simulink model "Hardware_Code"  (R2025b)
settings: Solver=FixedStepAuto  StartTime=0.0  StopTime=30  RelTol=1e-3  EnableMultiTasking=on
InitFcn:
  | battery_init;
  | Full_Charge_Volt=4.2; % unit volts
  | Cutoff_Volt=3; % unit volts
  | Delta=.02;
  | ContactorTime=20;
  | ContactorTimeOut=100;
  | High_TempLim=333;
  | Low_TempLim=253;
  | Sensor_Fault_Treshold=.02;
  | CurrentTimeout=1;
  | Allowed_Delta=.04;
  | Bal_On_Time=30;
  | Bal_Off_Time=5;
  | BalNotAct_Time=10;
values from neighbouring files (symbols this model uses):
  Charge_Rate = 1    [battery_init.m]
  Discharge_Rate = -1    [battery_init.m]
  Fly_Cycle_Current = [ ... (first row only)    [battery_init.m]
undefined symbols (not defined in the file or in its folder): batt, From_Plant_MATLABStruct, SRE
libraries: fl_lib x69, nesl_utility x54, ee_lib x12, batteryecm_lib x12, simulink x6, BatteryCurrentManagement x1
(part 1 of 2)
settings Model: DataDictionary=Needed_Buses.sldd  Creator=Odonata-KJ  LastModifiedBy=Odonata-KJ
settings OptimizationCC: DefaultParameterBehavior=Inlined  EnhancedBackFolding=on  PassReuseOutputArgsAs=Individual arguments  ZeroExternalMemoryAtStartup=off  ZeroInternalMemoryAtStartup=off  MaxStackSize=64  OptimizeBlockOrder=speed  DifferentSizesBufferReuse=on  OptimizationCustomize=off  EfficientTunableParamExpr=on
settings DebuggingCC: ParameterPrecisionLossMsg=none  ParameterTunabilityLossMsg=error  BusObjectLabelMismatch=none
settings HardwareCC: ProdBitPerPointer=32.0  ProdBitPerSizeT=32.0  ProdBitPerPtrDiffT=32.0  ProdLargestAtomicInteger=Long  ProdLargestAtomicFloat=Double  ProdWordSize=32.0  ProdLongLongMode=on  ProdHWDeviceType=ARM Compatible->ARM Cortex-M
settings SFSimCC: MATLABDynamicMemAlloc=off
settings RTWCC: SystemTargetFile=ert.tlc  HardwareBoard=STM32F4xx Based  TemplateMakefile=ert_default_tmf  Toolchain=GNU Tools for ARM Embedded Processors  Description=Embedded Coder
settings CodeAppCC: ForceParamTrailComments=on  IgnoreCustomStorageClasses=off  OperatorAnnotations=on  SimulinkDataObjDesc=on  SFDataObjDesc=on  InsertBlockDesc=on
settings ERTTargetCC: ExtModeTransport=3.0  ExtModeStaticAlloc=on  ExtModeStaticAllocSize=2048.0  ExtModeMexFile=ext_xcp  ExtModeIntrfLevel=Level2 - Open  TargetLangStandard=C99 (ISO)  CodeReplacementLibrary=ARM Cortex-M

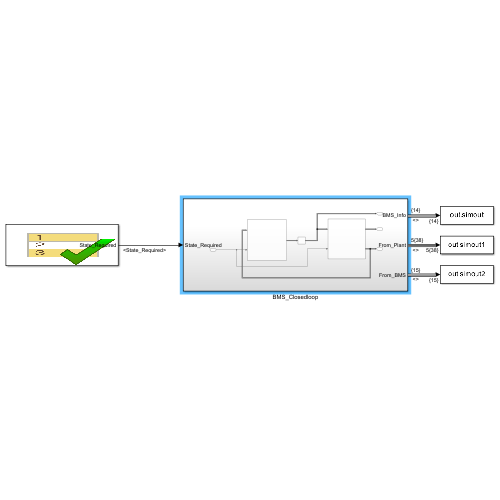
[thumbnail: Simulink's stored preview of the top-level diagram]
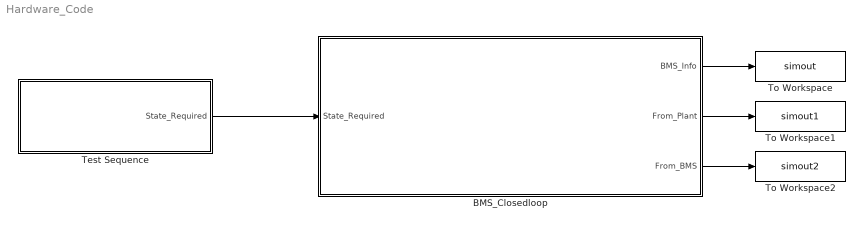
== system Hardware_Code ==
  BMS_Closedloop : Subsystem
  Test Sequence : Test Sequence  TreatAsAtomicUnit=on
  To Workspace : ToWorkspace  VariableName=simout  SaveFormat=Timeseries  SampleTime=-1
  To Workspace1 : ToWorkspace  VariableName=simout1  SaveFormat=Timeseries  SampleTime=-1
  To Workspace2 : ToWorkspace  VariableName=simout2  SaveFormat=Timeseries  SampleTime=-1
  wires:
  Test Sequence/1(State_Required) -> BMS_Closedloop/1(State_Required)
  BMS_Closedloop/1(BMS_Info) -> To Workspace/1
  BMS_Closedloop/2(From_Plant) -> To Workspace1/1
  BMS_Closedloop/3(From_BMS) -> To Workspace2/1

== system Hardware_Code/BMS_Closedloop ==
  State_Required : Inport
  BMS_Control : Subsystem
  Plant : Subsystem
  Unit Delay1 : UnitDelay  InitialCondition=From_Plant_MATLABStruct  SampleTime=-1  HasFrameUpgradeWarning=on
  BMS_Info : Outport
  From_Plant : Outport  Port=2
  From_BMS : Outport  Port=3
  wires:
  BMS_Control/1(BMS_Info) -> BMS_Info/1
  State_Required/1 -> BMS_Control/2(State_Required), Plant/2(State_Required)
  Plant/1(From_Plant) -> Unit Delay1/1
  BMS_Control/2(From_BMS) -> Plant/1(From_BMS), From_BMS/1
  Unit Delay1/1 -> From_Plant/1, BMS_Control/1(From_Plant)

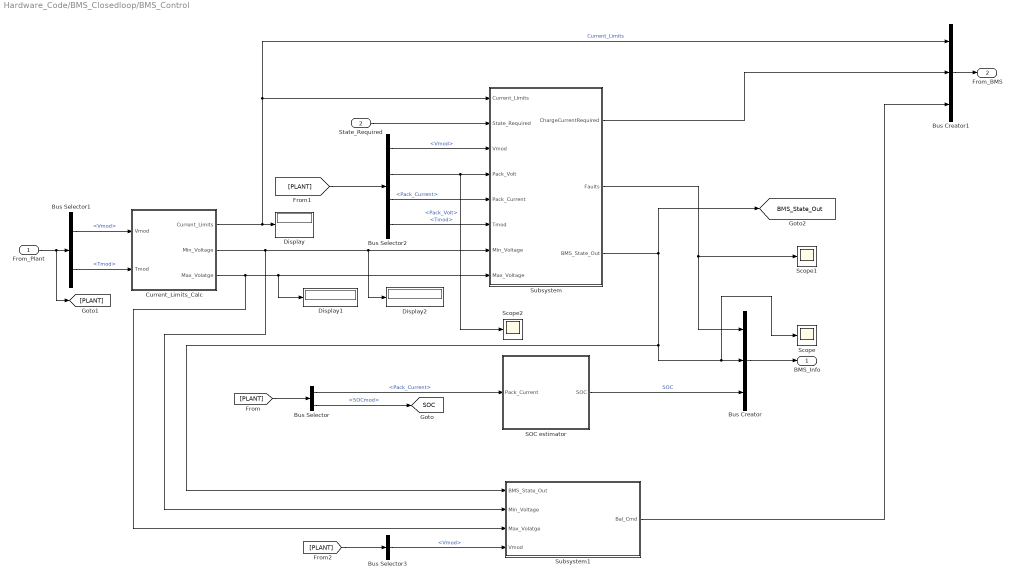
== system Hardware_Code/BMS_Closedloop/BMS_Control ==
  From_Plant : Inport
  State_Required : Inport  Port=2
  Bus Creator : BusCreator  Inputs=3
  Bus Creator1 : BusCreator  Inputs=3
  Bus Selector : BusSelector  OutputSignals=Pack_Current,SOCmod
  Bus Selector1 : BusSelector  OutputSignals=Vmod,Tmod
  Bus Selector2 : BusSelector  OutputSignals=Vmod,Pack_Volt,Pack_Current,Tmod
  Bus Selector3 : BusSelector  OutputSignals=Vmod
  Current_Limits_Calc : Subsystem
  Display : Display
  Display1 : Display
  Display2 : Display
  SOC estimator : Subsystem
  Scope : Scope
      settings: ActiveDisplayYMinimum=-0.83098117909981006  ActiveDisplayYMaximum=3.72716725840019  DataLoggingVariableName=ScopeData6
  Scope1 : Scope
      settings: ActiveDisplayYMinimum=-2.061290929652265  ActiveDisplayYMaximum=1.5304217223919956  DataLoggingVariableName=ScopeData7
  Scope2 : Scope
      settings: ActiveDisplayYMinimum=-21.052574610728009  ActiveDisplayYMaximum=61.397323890688391  DataLoggingVariableName=ScopeData8
  Subsystem : Subsystem
  Subsystem1 : Subsystem
  BMS_Info : Outport
  From_BMS : Outport  Port=2
  tag scope: BMS_State_Out=global, SOC=global
  wires:
  From_Plant/1 -> [PLANT], Bus Selector1/1
  [PLANT] -> Bus Selector/1
  Bus Selector1/1 -> Current_Limits_Calc/1(Vmod)  "<Vmod>"
  Current_Limits_Calc/2(Min_Voltage) -> Display2/1, Subsystem/7(Min_Voltage), Subsystem1/2(Min_Voltage)
  Current_Limits_Calc/3(Max_Volatge) -> Subsystem/8(Max_Voltage), Display1/1, Subsystem1/3(Max_Volatge)
  Current_Limits_Calc/1(Current_Limits) -> Subsystem/1(Current_Limits), Bus Creator1/1, Display/1  "Current_Limits"
  State_Required/1 -> Subsystem/2(State_Required)
  SOC estimator/1(SOC) -> Bus Creator/3  "SOC"
  Bus Creator/1 -> BMS_Info/1
  [PLANT] -> Bus Selector2/1
  Bus Creator1/1 -> From_BMS/1
  Subsystem/1(ChargeCurrentRequired) -> Bus Creator1/2
  Subsystem/2(Faults) -> Scope1/1, Bus Creator/1
  Subsystem/3(BMS_State_Out) -> [BMS_State_Out], Subsystem1/1(BMS_State_Out), Scope/1, Bus Creator/2
  [PLANT] -> Bus Selector3/1
  Bus Selector3/1 -> Subsystem1/4(Vmod)  "<Vmod>"
  Subsystem1/1(Bal_Cmd) -> Bus Creator1/3
  Bus Selector/1 -> SOC estimator/1(Pack_Current)  "<Pack_Current>"
  Bus Selector/2 -> [SOC]  "<SOCmod>"
  Bus Selector2/1 -> Subsystem/3(Vmod)  "<Vmod>"
  Bus Selector2/4 -> Subsystem/6(Tmod)  "<Tmod>"
  Bus Selector2/2 -> Scope2/1, Subsystem/4(Pack_Volt)  "<Pack_Volt>"
  Bus Selector2/3 -> Subsystem/5(Pack_Current)  "<Pack_Current>"
  Bus Selector1/2 -> Current_Limits_Calc/2(Tmod)  "<Tmod>"

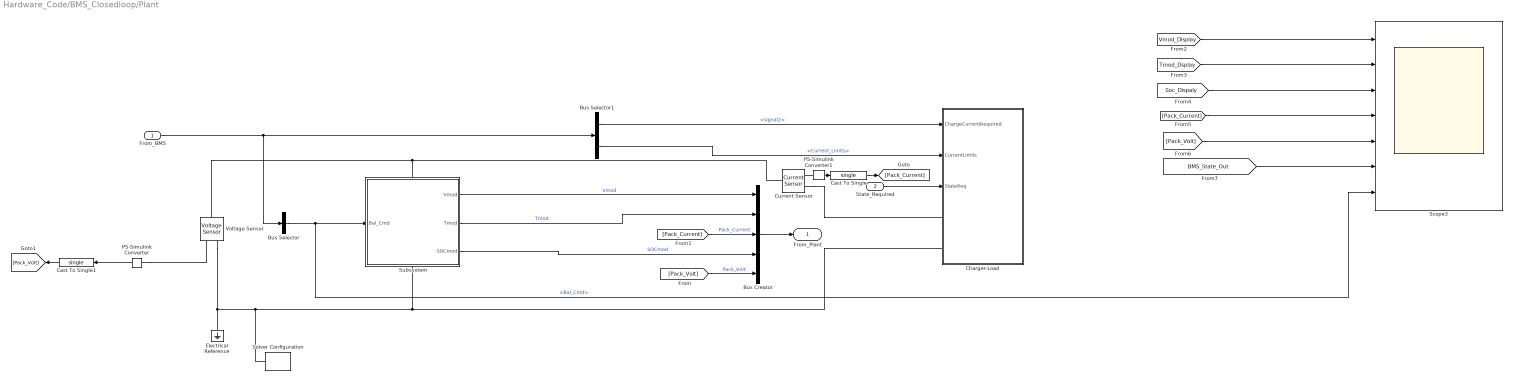
== system Hardware_Code/BMS_Closedloop/Plant ==
  From_BMS : Inport
  State_Required : Inport  Port=2
  Bus Creator : BusCreator  Inputs=5
  Bus Selector : BusSelector  OutputSignals=Bal_Cmd
  Bus Selector1 : BusSelector  OutputSignals=signal2,Current_Limits
  Cast To Single : DataTypeConversion  OutDataTypeStr=single  SaturateOnIntegerOverflow=off  RndMeth=Floor
  Cast To Single1 : DataTypeConversion  OutDataTypeStr=single  SaturateOnIntegerOverflow=off  RndMeth=Floor
  Charger-Load : Subsystem
  Current Sensor : fl_lib/Electrical/Electrical Sensors/Current Sensor
  Electrical Reference : fl_lib/Electrical/Electrical Elements/Electrical Reference
  PS-Simulink Converter : nesl_utility/PS-Simulink Converter  PhysicalDomain=network_engine_domain  SubClassName=ps_output  LeftPortType=input  RightPortType=output  PseudoPeriodic=off  Frequencies=[]  VectorFormat=inherit  Unit=inherit  AffineConversion=off
  PS-Simulink Converter1 : nesl_utility/PS-Simulink Converter  PhysicalDomain=network_engine_domain  SubClassName=ps_output  LeftPortType=input  RightPortType=output  PseudoPeriodic=off  Frequencies=[]  VectorFormat=inherit  Unit=inherit  AffineConversion=off
  Scope3 : Scope  NumInputPorts=7
      settings: ActiveDisplayString=5  ActiveDisplayYMinimum=32.848355293273926  ActiveDisplayYMaximum=53.971850395202637  YLabel=Pack Volt  DataLoggingVariableName=ScopeData10
  Solver Configuration : nesl_utility/Solver Configuration  PhysicalDomain=network_engine_domain  SubClassName=solver  LeftPortType=input  RightPortType=generic  Tones=[]  Harmonics=[]  SimulateNoise=off  Profile=off  UseLocalSampling=off  EnableSwitchedLinearOptims=on  FrequencyDomain=off  UseCCode=off  RelTol=0.001  AbsTol=0.001  MinStep=1e-09  ToWorkspace=off  RevertToSquareIcSolve=off  NumHomotopyIterations=100  PhasorMode=off  PhasorModeNumHarmonics=1  ConsistencySolver=NEWTON_XTOL_AFTER_FTOL  IndexReductionMethod=DerivativeReplacement  DoDC=off  ResidualTolerance=1e-09  ConsistencyTolSource=GLOBAL  ConsistencyAbsTol=0.001  ConsistencyRelTol=0.001  ConsistencyTolFactor=0.001  UseLocalSolver=on  LocalSolverChoice=NE_BACKWARD_EULER_ADVANCER  ResolveIndetEquations=on  FunctionEvalNumThread=1  LocalSolverSampleTime=0.001  DoFixedCost=off  MaxNonlinIter=3  MaxModeIter=2  ComputeImpulses=off  ImpulseIterations=2  LinearAlgebra=auto  LinearAlgebraNumThread=0  EquationFormulation=NE_TIME_EF  DelaysMemoryBudget=1024  AutomaticFiltering=on  FilteringTimeConstant=0.001  PartitionStorageMethod=AS_NEEDED  PartitionMemoryBudget=1024  PartitionMethod=ROBUST  MultibodyUseLocalSolver=off  MultibodyLocalSolverChoice=ODE1  MultibodyLocalSolverSampleTime=0.001
  Subsystem : Subsystem
      settings: PortSchema="{\"entries\":[{\"content\":{\"sides\":[{\"content\":{\"connectorIds\":[\"In1\"]},\"type\":\"ConnectorPlacement.EquallySpacedRectSide\",\"uuid\":\"58357de5-60ff-42e3-841b-e50425142caf\"},{\"content\":{\"connectorIds\":[\"Out1\",\"Out2\",\"Out3\"],\"side\":\"RIGHT\"},\"type\":\"ConnectorPlacement.EquallySpacedRectSide\",\"uuid\":\"e2d7d04f-a8ca-435a-9027-c1ea19fe7b57\"},{\"content\":{\"connectorIds\":[\"LConn1\"],\"side\":\"TOP\"},\"type\":\"ConnectorPlacement.EquallySpacedRectSide\",\"uuid\":\"61bcd3f6-6975-41f2-a4de-83d930262737\"},{\"content\":{\"connectorIds\":[\"RConn1\"],\"side\":\"BOTTOM\"},\"type\":\"ConnectorPlacement.EquallySpacedRectSide\",\"uuid\":\"f64ac1d4-74b0-46a5-b79a-ed01bae0794c\"}]},\"type\":\"ConnectorPlacement.EquallySpacedConnector\",\"uuid\":\"11abc81f-2488-49dd-a311-a0e5e9bbc669\"}],\"packageUris\":[\"http://schema.mathworks.com/mf0/Connector/R2020b\"],\"version\":\"1.0\"}"
  Voltage Sensor : fl_lib/Electrical/Electrical Sensors/Voltage Sensor
  From_Plant : Outport
  wires:
  Bus Creator/1 -> From_Plant/1
  Subsystem/1(Vmod) -> Bus Creator/1  "Vmod"
  Subsystem/2(Tmod) -> Bus Creator/2  "Tmod"
  PS-Simulink Converter/1 -> Cast To Single1/1
  [Pack_Volt] -> Bus Creator/5  "Pack_Volt"
  From_BMS/1 -> Bus Selector/1, Bus Selector1/1
  State_Required/1 -> Charger-Load/3(StateReq)
  Bus Selector1/1 -> Charger-Load/1(ChargeCurrentRequired)  "<signal2>"
  Bus Selector1/2 -> Charger-Load/2(CurrentLimits)  "<Current_Limits>"
  Bus Selector/1 -> Scope3/7, Subsystem/1(Bal_Cmd)  "<Bal_Cmd>"
  Subsystem/3(SOCmod) -> Bus Creator/4  "SOCmod"
  PS-Simulink Converter1/1 -> Cast To Single/1
  [Pack_Current] -> Bus Creator/3  "Pack_Current"
  Cast To Single/1 -> [Pack_Current]
  Cast To Single1/1 -> [Pack_Volt]
  [Vmod_Display] -> Scope3/1
  [Tmod_Dsplay] -> Scope3/2
  [Soc_Dispaly] -> Scope3/3
  [Pack_Current] -> Scope3/4
  [Pack_Volt] -> Scope3/5
  [BMS_State_Out] -> Scope3/6
  connections:
  Current Sensor/LConn1 -- Subsystem/LConn1 -- Voltage Sensor/LConn1
  Voltage Sensor/RConn2 -- Electrical Reference/LConn1 -- Solver Configuration/RConn1 -- Charger-Load/LConn2 -- Subsystem/RConn1
  PS-Simulink Converter/LConn1 -- Voltage Sensor/RConn1
  Current Sensor/RConn2 -- Charger-Load/LConn1
  PS-Simulink Converter1/LConn1 -- Current Sensor/RConn1

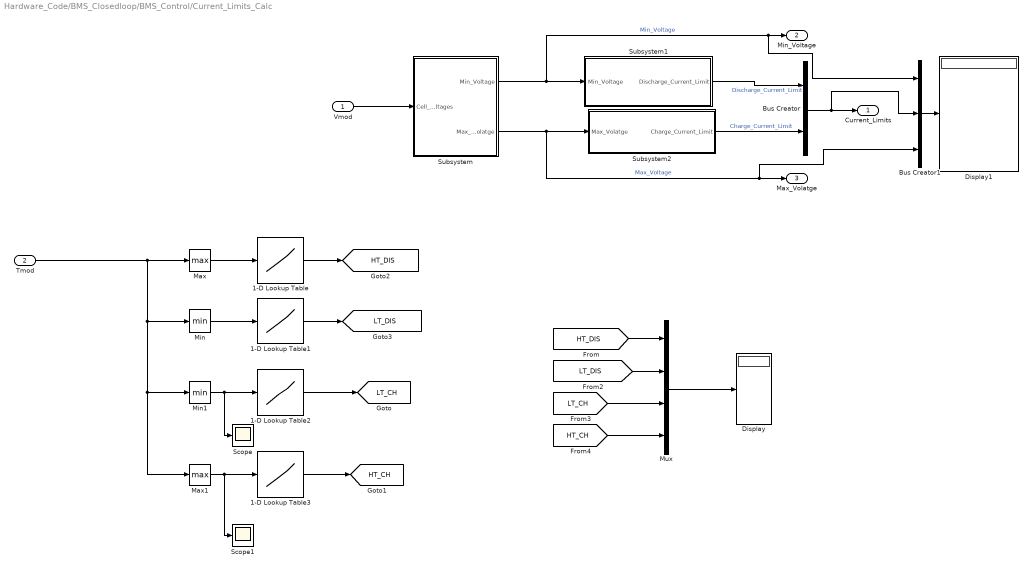
== system Hardware_Code/BMS_Closedloop/BMS_Control/Current_Limits_Calc ==
  Vmod : Inport
  Tmod : Inport  Port=2
  1-D Lookup Table : Lookup_n-D  NumberOfTableDimensions=1  BreakpointsForDimension1=[296.15;313.15;333.15]  Table=[25;24;23]  InternalRulePriority=Speed  RndMeth=Simplest
  1-D Lookup Table1 : Lookup_n-D  NumberOfTableDimensions=1  BreakpointsForDimension1=[253.15 263.15 273.15]  Table=[16 21 21]  InternalRulePriority=Speed  RndMeth=Simplest
  1-D Lookup Table2 : Lookup_n-D  NumberOfTableDimensions=1  BreakpointsForDimension1=[253.15 263.15 273.15]  Table=[0 0 .5]  InternalRulePriority=Speed  RndMeth=Simplest
  1-D Lookup Table3 : Lookup_n-D  NumberOfTableDimensions=1  BreakpointsForDimension1=[278.15 283.15 298.15 313.15 318.15 323.15]  Table=[1.5 3 6 4 2 0]  InternalRulePriority=Speed  RndMeth=Simplest
  Bus Creator : BusCreator  Inputs=2
  Bus Creator1 : BusCreator  Inputs=3
  Display : Display
  Display1 : Display
  Max : MinMax  Function=max
  Max1 : MinMax  Function=max
  Min : MinMax
  Min1 : MinMax
  Mux : Mux
  Scope : Scope
      settings: ActiveDisplayYMinimum=-0.8873535688334071  ActiveDisplayYMaximum=0.8403216282295447  DataLoggingVariableName=ScopeData16
  Scope1 : Scope
      settings: ActiveDisplayYMinimum=-1  ActiveDisplayYMaximum=1  DataLoggingVariableName=ScopeData17
  Subsystem : Subsystem
  Subsystem1 : Subsystem
  Subsystem2 : Subsystem
  Current_Limits : Outport
  Min_Voltage : Outport  Port=2
  Max_Volatge : Outport  Port=3
  tag scope: HT_CH=global, HT_DIS=global, LT_CH=global, LT_DIS=global
  wires:
  Vmod/1 -> Subsystem/1(Cell_Voltages)
  Subsystem/1(Min_Voltage) -> Bus Creator1/1, Min_Voltage/1, Subsystem1/1(Min_Voltage)  "Min_Voltage"
  Max/1 -> 1-D Lookup Table/1
  Tmod/1 -> Max/1, Min/1, Min1/1, Max1/1
  Min/1 -> 1-D Lookup Table1/1
  1-D Lookup Table1/1 -> [LT_DIS]
  1-D Lookup Table/1 -> [HT_DIS]
  Subsystem/2(Max_Volatge) -> Bus Creator1/3, Max_Volatge/1, Subsystem2/1(Max_Volatge)  "Max_Voltage"
  Min1/1 -> Scope/1, 1-D Lookup Table2/1
  Max1/1 -> Scope1/1, 1-D Lookup Table3/1
  1-D Lookup Table2/1 -> [LT_CH]
  1-D Lookup Table3/1 -> [HT_CH]
  Mux/1 -> Display/1
  [HT_DIS] -> Mux/1
  [LT_DIS] -> Mux/2
  [LT_CH] -> Mux/3
  [HT_CH] -> Mux/4
  Subsystem1/1(Discharge_Current_Limit) -> Bus Creator/1  "Discharge_Current_Limit"
  Subsystem2/1(Charge_Current_Limit) -> Bus Creator/2  "Charge_Current_Limit"
  Bus Creator/1 -> Bus Creator1/2, Current_Limits/1
  Bus Creator1/1 -> Display1/1

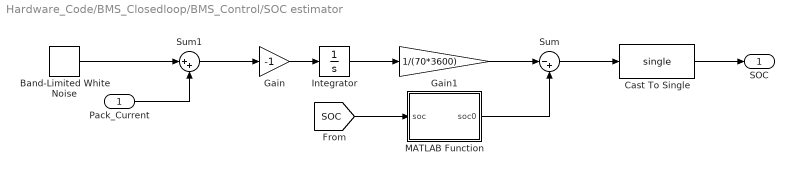
== system Hardware_Code/BMS_Closedloop/BMS_Control/SOC estimator ==
  Pack_Current : Inport
  Band-Limited White Noise : simulink/Sources/Band-Limited White Noise  Cov=[0.1]  Ts=.001  seed=[23341]
  Cast To Single : DataTypeConversion  OutDataTypeStr=single  SaturateOnIntegerOverflow=off  RndMeth=Floor
  Gain : Gain  Gain=-1
  Gain1 : Gain  Gain=1/(70*3600)
  Integrator : Integrator
  MATLAB Function : MATLAB Function  TreatAsAtomicUnit=on
  Sum : Sum  Inputs=|-+
  Sum1 : Sum  Inputs=|++
  SOC : Outport
  wires:
  Gain/1 -> Integrator/1
  Integrator/1 -> Gain1/1
  [SOC] -> MATLAB Function/1(soc)
  Gain1/1 -> Sum/1
  MATLAB Function/1(soc0) -> Sum/2
  Sum/1 -> Cast To Single/1
  Sum1/1 -> Gain/1
  Band-Limited White Noise/1 -> Sum1/1
  Pack_Current/1 -> Sum1/2
  Cast To Single/1 -> SOC/1

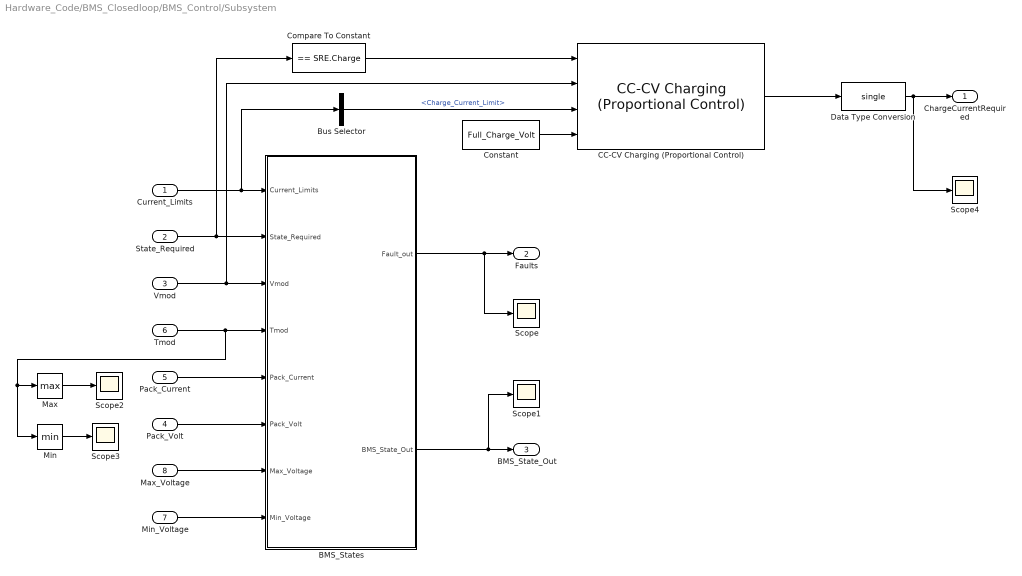
== system Hardware_Code/BMS_Closedloop/BMS_Control/Subsystem ==
  Current_Limits : Inport
  State_Required : Inport  Port=2
  Vmod : Inport  Port=3
  Pack_Volt : Inport  Port=4  OutDataTypeStr=single
  Pack_Current : Inport  Port=5  OutDataTypeStr=single
  Tmod : Inport  Port=6
  Min_Voltage : Inport  Port=7
  Max_Voltage : Inport  Port=8
  BMS_States : Stateflow chart  TreatAsAtomicUnit=on
      settings: PortSchema="{\"entries\":[{\"content\":{\"sides\":[{\"content\":{\"connectorIds\":[\"In1\",\"In6\",\"In2\",\"In3\",\"In4\",\"In5\",\"In7\",\"In8\"]},\"type\":\"ConnectorPlacement.EquallySpacedRectSide\",\"uuid\":\"75752650-a65f-4df2-8429-36d8f2b8ac99\"},{\"content\":{\"connectorIds\":[\"Out1\",\"Out2\"],\"side\":\"RIGHT\"},\"type\":\"ConnectorPlacement.EquallySpacedRectSide\",\"uuid\":\"5c64a1aa-fdb2-4c0c-b2ff-5c47ddc01ea2\"},{\"content\":{\"side\":\"TOP\"},\"type\":\"ConnectorPlacement.EquallySpacedRectSide\",\"uuid\":\"c92e07e0-a1c3-44d4-87a0-5a0cb4ce56f3\"}]},\"type\":\"ConnectorPlacement.EquallySpacedConnector\",\"uuid\":\"9d97857d-a16c-4ff3-995b-4c10703be4f7\"}],\"packageUris\":[\"http://schema.mathworks.com/mf0/Connector/R2020b\"],\"version\":\"1.0\"}"
  Bus Selector : BusSelector  OutputSignals=Charge_Current_Limit
  CC-CV Charging (Proportional Control) : BatteryCurrentManagement/CC-CV Charging (Proportional Control)  MinMaxFlag=off  Kp=0.02  Ts=.001
      settings: LibrarySourceBlock=batt_sl_lib/Current Management/CC-CV Charging (Proportional Control)
  Compare To Constant : simulink/Logic and Bit Operations/Compare To Constant  relop===  const=SRE.Charge  OutDataTypeStr=boolean
  Constant : Constant  Value=Full_Charge_Volt
  Data Type Conversion : DataTypeConversion  OutDataTypeStr=single  SaturateOnIntegerOverflow=off  RndMeth=Floor
  Max : MinMax  Function=max
  Min : MinMax
  Scope{,1..4} (5 alike) : Scope
      Scope settings: ActiveDisplayYMinimum=-22.268675590472341  ActiveDisplayYMaximum=16.214223204352443
      Scope1 settings: ActiveDisplayYMinimum=-5.7492294138692648  ActiveDisplayYMaximum=5.5777504485478211
      Scope2 settings: ActiveDisplayYMinimum=228.00617188854886  ActiveDisplayYMaximum=391.56515067069523  DataLoggingVariableName=ScopeData3
      Scope3 settings: ActiveDisplayYMinimum=250.29214528704537  ActiveDisplayYMaximum=307.46054262836492  DataLoggingVariableName=ScopeData9
      Scope4 settings: ActiveDisplayYMinimum=-92.188124656677246  ActiveDisplayYMaximum=10.243124961853026  DataLoggingVariableName=ScopeData4
  ChargeCurrentRequired : Outport  OutDataTypeStr=single
  Faults : Outport  Port=2
  BMS_State_Out : Outport  Port=3
  wires:
  Vmod/1 -> BMS_States/2(Vmod), CC-CV Charging (Proportional Control)/2
  Tmod/1 -> Max/1, Min/1, BMS_States/3(Tmod)
  Pack_Current/1 -> BMS_States/4(Pack_Current)
  Pack_Volt/1 -> BMS_States/5(Pack_Volt)
  Max_Voltage/1 -> BMS_States/7(Max_Voltage)
  Min_Voltage/1 -> BMS_States/8(Min_Voltage)
  State_Required/1 -> Compare To Constant/1, BMS_States/6(State_Required)
  Current_Limits/1 -> Bus Selector/1, BMS_States/1(Current_Limits)
  Constant/1 -> CC-CV Charging (Proportional Control)/4
  CC-CV Charging (Proportional Control)/1 -> Data Type Conversion/1
  BMS_States/1(Fault_out) -> Scope/1, Faults/1
  Compare To Constant/1 -> CC-CV Charging (Proportional Control)/1
  BMS_States/2(BMS_State_Out) -> Scope1/1, BMS_State_Out/1
  Bus Selector/1 -> CC-CV Charging (Proportional Control)/3  "<Charge_Current_Limit>"
  Max/1 -> Scope2/1
  Data Type Conversion/1 -> ChargeCurrentRequired/1, Scope4/1
  Min/1 -> Scope3/1

== system Hardware_Code/BMS_Closedloop/BMS_Control/Subsystem1 ==
  BMS_State_Out : Inport
  Min_Voltage : Inport  Port=2
  Max_Volatge : Inport  Port=3
  Vmod : Inport  Port=4
  Chart : Stateflow chart  TreatAsAtomicUnit=on
  Bal_Cmd : Outport
  wires:
  BMS_State_Out/1 -> Chart/1(BMS_State_Out)
  Min_Voltage/1 -> Chart/2(Min_Voltage)
  Chart/1(Bal_Cmd) -> Bal_Cmd/1
  Vmod/1 -> Chart/4(Vmod)
  Max_Volatge/1 -> Chart/3(Max_Voltage)

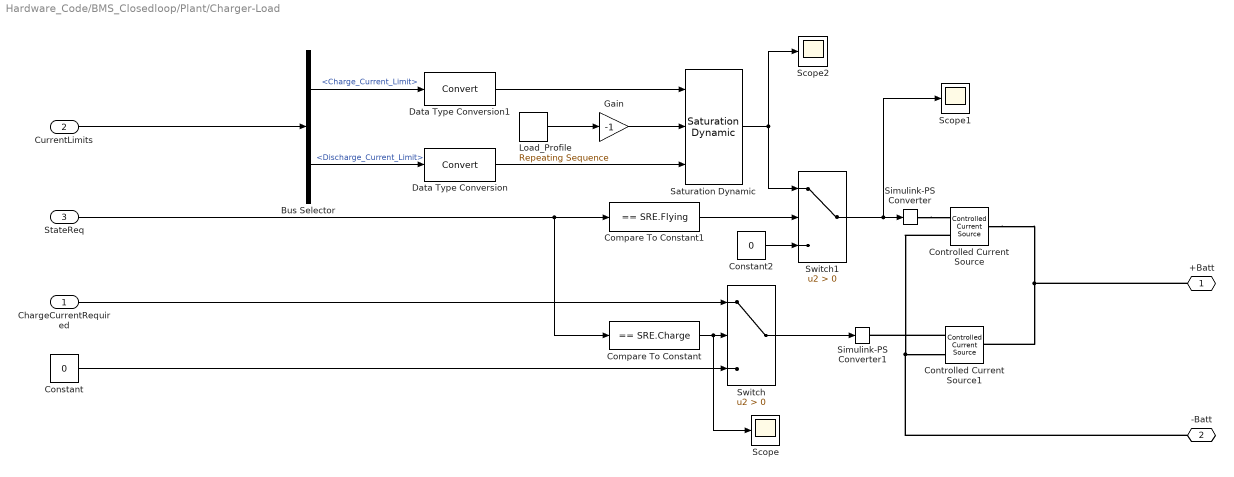
== system Hardware_Code/BMS_Closedloop/Plant/Charger-Load ==
  ChargeCurrentRequired : Inport
  CurrentLimits : Inport  Port=2
  StateReq : Inport  Port=3
  Bus Selector : BusSelector  OutputSignals=Charge_Current_Limit,Discharge_Current_Limit
  Compare To Constant : simulink/Logic and Bit Operations/Compare To Constant  relop===  const=SRE.Charge  OutDataTypeStr=boolean
  Compare To Constant1 : simulink/Logic and Bit Operations/Compare To Constant  relop===  const=SRE.Flying  OutDataTypeStr=boolean
  Constant : Constant  Value=0
  Constant2 : Constant  Value=0
  Controlled Current Source : fl_lib/Electrical/Electrical Sources/Controlled Current Source
  Controlled Current Source1 : fl_lib/Electrical/Electrical Sources/Controlled Current Source
  Data Type Conversion : DataTypeConversion  SaturateOnIntegerOverflow=off  RndMeth=Floor
  Data Type Conversion1 : DataTypeConversion  SaturateOnIntegerOverflow=off  RndMeth=Floor
  Gain : Gain  Gain=-1
  Load_Profile : simulink/Sources/Repeating Sequence  rep_seq_t=Fly_Cycle_Current (:,1)  rep_seq_y=Fly_Cycle_Current (:,2)
  Saturation Dynamic : simulink/Discontinuities/Saturation Dynamic  OutMin=[]  OutMax=[]  OutDataTypeStr=Inherit: Same as second input  OutDataType=fixdt(1, 16)  OutScaling=2^-10  DoSatur=off
  Scope : Scope
      settings: ActiveDisplayYMinimum=-1  ActiveDisplayYMaximum=1  DataLoggingVariableName=ScopeData2
  Scope1 : Scope
      settings: ActiveDisplayYMinimum=-1  ActiveDisplayYMaximum=1  DataLoggingVariableName=ScopeData5
  Scope2 : Scope
      settings: ActiveDisplayYMinimum=-103.02204279771105  ActiveDisplayYMaximum=6.6759845742817987  DataLoggingVariableName=ScopeData11
  Simulink-PS Converter : nesl_utility/Simulink-PS Converter  PhysicalDomain=network_engine_domain  SubClassName=ps_input  LeftPortType=input  RightPortType=output  PseudoPeriodic=off  Frequencies=[]  NoiseDistribution=none  NoiseParameters=[]  Unit=1  AffineConversion=off  FilteringAndDerivatives=provide  SimscapeFilterOrder=1  InputFilterTimeConstant=0.001  UdotUserProvided=0
  Simulink-PS Converter1 : nesl_utility/Simulink-PS Converter  PhysicalDomain=network_engine_domain  SubClassName=ps_input  LeftPortType=input  RightPortType=output  PseudoPeriodic=off  Frequencies=[]  NoiseDistribution=none  NoiseParameters=[]  Unit=1  AffineConversion=off  FilteringAndDerivatives=provide  SimscapeFilterOrder=1  InputFilterTimeConstant=0.001  UdotUserProvided=0
  Switch : Switch  Criteria=u2 > Threshold  SaturateOnIntegerOverflow=off  InputSameDT=off
  Switch1 : Switch  Criteria=u2 > Threshold  SaturateOnIntegerOverflow=off  InputSameDT=off
  +Batt : PMIOPort  Side=Left
  -Batt : PMIOPort  Port=2  Side=Left
  wires:
  StateReq/1 -> Compare To Constant/1, Compare To Constant1/1
  Compare To Constant/1 -> Scope/1, Switch/2
  Switch/1 -> Simulink-PS Converter1/1
  CurrentLimits/1 -> Bus Selector/1
  Gain/1 -> Saturation Dynamic/2
  Switch1/1 -> Scope1/1, Simulink-PS Converter/1
  Saturation Dynamic/1 -> Switch1/1, Scope2/1
  Compare To Constant1/1 -> Switch1/2
  Constant2/1 -> Switch1/3
  Bus Selector/1 -> Data Type Conversion1/1  "<Charge_Current_Limit>"
  Bus Selector/2 -> Data Type Conversion/1  "<Discharge_Current_Limit>"
  Data Type Conversion/1 -> Saturation Dynamic/3
  Data Type Conversion1/1 -> Saturation Dynamic/1
  Constant/1 -> Switch/3
  ChargeCurrentRequired/1 -> Switch/1
  Load_Profile/1 -> Gain/1
  connections:
  Simulink-PS Converter/RConn1 -- Controlled Current Source/RConn1
  Controlled Current Source1/RConn1 -- Simulink-PS Converter1/RConn1
  +Batt/RConn1 -- Controlled Current Source1/LConn1 -- Controlled Current Source/LConn1
  -Batt/RConn1 -- Controlled Current Source/RConn2 -- Controlled Current Source1/RConn2

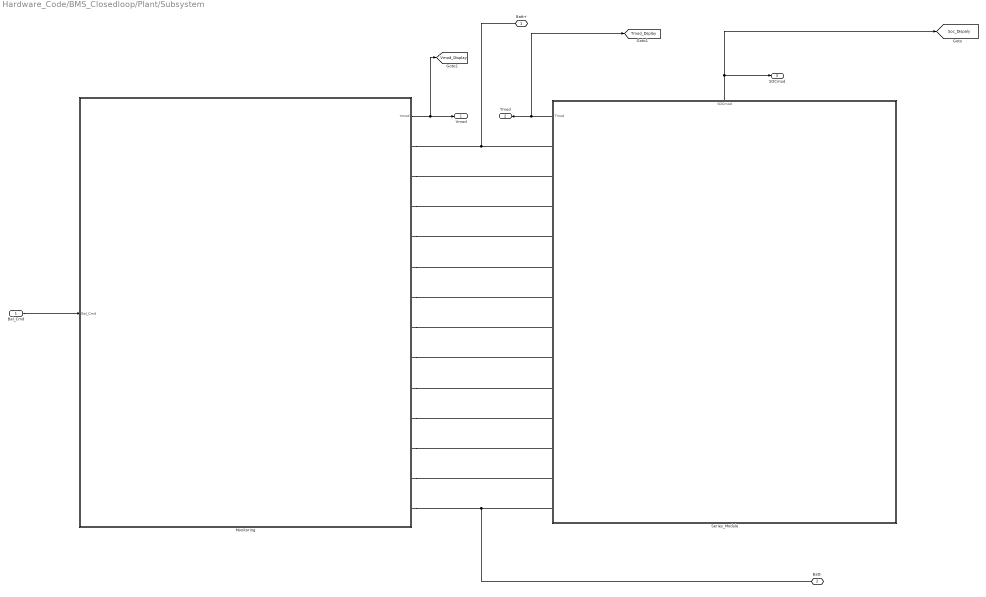
== system Hardware_Code/BMS_Closedloop/Plant/Subsystem ==
  Bal_Cmd : Inport  OutDataTypeStr=boolean
  Monitoring : Subsystem
  Series_Module : Subsystem
      settings: PortSchema="{\"entries\":[{\"content\":{\"sides\":[{\"content\":{\"connectorIds\":[\"Out2\",\"LConn1\",\"LConn2\",\"LConn3\",\"LConn4\",\"LConn5\",\"LConn6\",\"LConn7\",\"LConn8\",\"LConn9\",\"LConn10\",\"LConn11\",\"LConn12\",\"LConn13\"]},\"type\":\"ConnectorPlacement.EquallySpacedRectSide\",\"uuid\":\"c6d0ec2f-e215-49aa-88c4-aa36f54ff2d8\"},{\"content\":{\"side\":\"RIGHT\"},\"type\":\"ConnectorPlacement.EquallySpacedRectSide\",\"uuid\":\"ce965262-80da-4022-87ce-2d028a90e212\"},{\"content\":{\"connectorIds\":[\"Out1\"],\"side\":\"TOP\"},\"type\":\"ConnectorPlacement.EquallySpacedRectSide\",\"uuid\":\"06d9cb93-079f-49de-a983-b6840e947914\"}]},\"type\":\"ConnectorPlacement.EquallySpacedConnector\",\"uuid\":\"29985f6b-b161-490b-875e-190c720c1d7b\"}],\"packageUris\":[\"http://schema.mathworks.com/mf0/Connector/R2020b\"],\"version\":\"1.0\"}"
  Batt+ : PMIOPort  Side=Left
  Batt- : PMIOPort  Port=2  Side=Right
  Vmod : Outport
  Tmod : Outport  Port=2
  SOCmod : Outport  Port=3
  tag scope: Soc_Dispaly=global, Tmod_Dsplay=global, Vmod_Display=global
  wires:
  Bal_Cmd/1 -> Monitoring/1(Bal_Cmd)
  Monitoring/1(Vmod) -> [Vmod_Display], Vmod/1
  Series_Module/2(Tmod) -> [Tmod_Dsplay], Tmod/1
  Series_Module/1(SOCmod) -> [Soc_Dispaly], SOCmod/1
  connections:
  Monitoring/RConn1 -- Series_Module/LConn1 -- Batt+/RConn1
  Monitoring/RConn2 -- Series_Module/LConn2
  Monitoring/RConn3 -- Series_Module/LConn3
  Monitoring/RConn4 -- Series_Module/LConn4
  Monitoring/RConn5 -- Series_Module/LConn5
  Monitoring/RConn6 -- Series_Module/LConn6
  Monitoring/RConn7 -- Series_Module/LConn7
  Monitoring/RConn8 -- Series_Module/LConn8
  Monitoring/RConn9 -- Series_Module/LConn9
  Monitoring/RConn10 -- Series_Module/LConn10
  Monitoring/RConn11 -- Series_Module/LConn11
  Monitoring/RConn12 -- Series_Module/LConn12
  Monitoring/RConn13 -- Batt-/RConn1 -- Series_Module/LConn13

== system Hardware_Code/BMS_Closedloop/BMS_Control/Current_Limits_Calc/Subsystem ==
  Cell_Voltages : Inport
  Max : MinMax  Function=max
  MinMax : MinMax
  Min_Voltage : Outport
  Max_Volatge : Outport  Port=2
  wires:
  Cell_Voltages/1 -> Max/1, MinMax/1
  MinMax/1 -> Min_Voltage/1
  Max/1 -> Max_Volatge/1

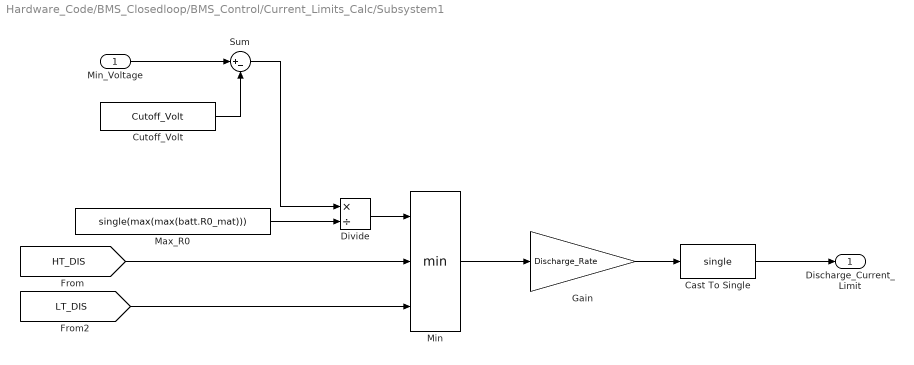
== system Hardware_Code/BMS_Closedloop/BMS_Control/Current_Limits_Calc/Subsystem1 ==
  Min_Voltage : Inport
  Cast To Single : DataTypeConversion  OutDataTypeStr=single  SaturateOnIntegerOverflow=off  RndMeth=Floor
  Cutoff_Volt : Constant  Value=Cutoff_Volt
  Divide : Product  Inputs=*/
  Gain : Gain  Gain=Discharge_Rate
  Max_R0 : Constant  Value=single(max(max(batt.R0_mat)))
  Min : MinMax  Inputs=3
  Sum : Sum  Inputs=|+-
  Discharge_Current_Limit : Outport
  wires:
  Min_Voltage/1 -> Sum/1
  Cutoff_Volt/1 -> Sum/2
  Sum/1 -> Divide/1
  Max_R0/1 -> Divide/2
  Divide/1 -> Min/1
  [HT_DIS] -> Min/2
  [LT_DIS] -> Min/3
  Min/1 -> Gain/1
  Cast To Single/1 -> Discharge_Current_Limit/1
  Gain/1 -> Cast To Single/1

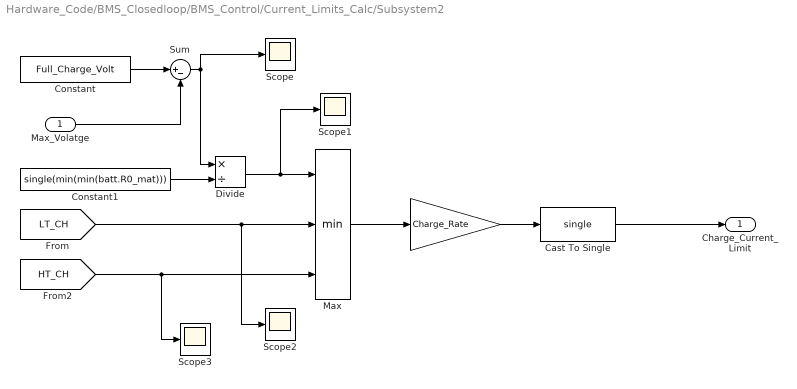
== system Hardware_Code/BMS_Closedloop/BMS_Control/Current_Limits_Calc/Subsystem2 ==
  Max_Volatge : Inport
  " " : Gain  Gain=Charge_Rate
  Cast To Single : DataTypeConversion  OutDataTypeStr=single  SaturateOnIntegerOverflow=off  RndMeth=Floor
  Constant : Constant  Value=Full_Charge_Volt
  Constant1 : Constant  Value=single(min(min(batt.R0_mat)))
  Divide : Product  Inputs=*/
  Max : MinMax  Inputs=3
  Scope{,1..3} (4 alike) : Scope
      Scope settings: ActiveDisplayYMinimum=-9.8962889072515861  ActiveDisplayYMaximum=7.3804630633779373  DataLoggingVariableName=ScopeData12
      Scope1 settings: ActiveDisplayYMinimum=-1  ActiveDisplayYMaximum=1  DataLoggingVariableName=ScopeData13
      Scope2 settings: ActiveDisplayYMinimum=-1  ActiveDisplayYMaximum=1  DataLoggingVariableName=ScopeData14
      Scope3 settings: ActiveDisplayYMinimum=-1  ActiveDisplayYMaximum=1  DataLoggingVariableName=ScopeData15
  Sum : Sum  Inputs=|+-
  Charge_Current_Limit : Outport
  wires:
  Constant/1 -> Sum/1
  Max_Volatge/1 -> Sum/2
  Sum/1 -> Divide/1, Scope/1
  Constant1/1 -> Divide/2
  Divide/1 -> Scope1/1, Max/1
  [LT_CH] -> Max/2, Scope2/1
  [HT_CH] -> Scope3/1, Max/3
  Max/1 -> " "/1
  Cast To Single/1 -> Charge_Current_Limit/1
  " "/1 -> Cast To Single/1

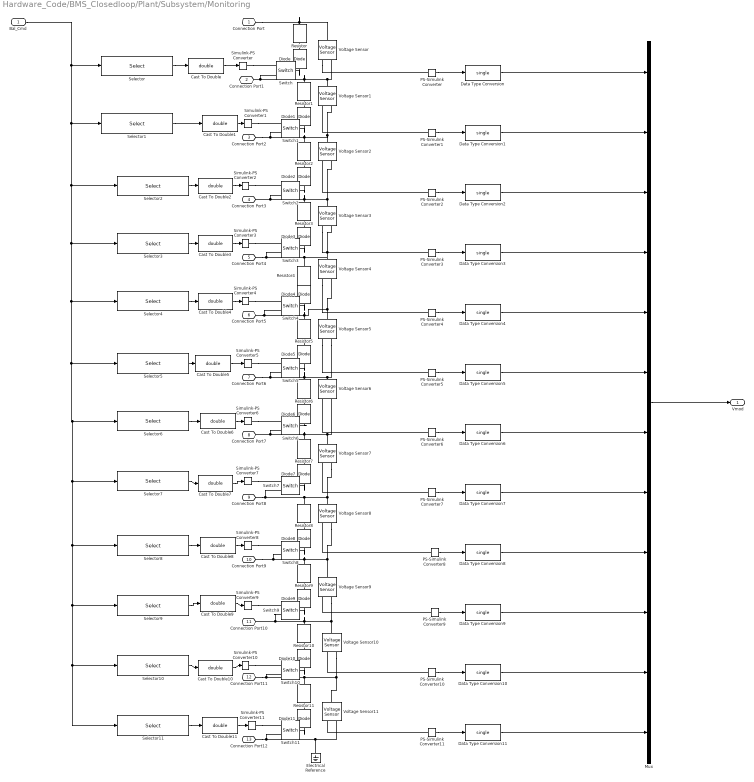
== system Hardware_Code/BMS_Closedloop/Plant/Subsystem/Monitoring ==
  Bal_Cmd : Inport  OutDataTypeStr=boolean
  Cast To Double{,1..11} (12 alike) : DataTypeConversion  OutDataTypeStr=double  SaturateOnIntegerOverflow=off  RndMeth=Floor
  Data Type Conversion{,1..11} (12 alike) : DataTypeConversion  OutDataTypeStr=single  SaturateOnIntegerOverflow=off  RndMeth=Floor
  Diode{,1..11} (12 alike) : ee_lib/Semiconductors & Converters/Diode  ModelType=ee.enum.diode.modelType.pwl  TableType=ee.enum.diode.tableType.IfMat  IfMat=[.07, .12, .19, 1.75, 4.24, 7.32, 11.2; .16, .3, .72, 2.14, 5.02, 8.35, 13.12] A  VfMat=[.9, 1.15, 1.25, 1.5, 1.75, 2.17, 2.6, 2.85; .58, .68, .75, 1.1, 1.38, 1.77, 2.27, 2.7] V  TjVec=[25, 125] degC  VfVec=[.5, .7, .9, 1.3, 1.7, 2.1, 2.5] V  IfVec=[.1, .2, .5, 1, 2, 4, 7, 10] A  IrMat=[1e-06, 2e-06, 5e-06, 1e-05, 2.5e-05, 5e-05, .0001; 2e-06, 5e-06, 1e-05, 4e-05, 8e-05, .0002, .0005] A  VrMat=[10, 100, 200, 250, 300, 325, 350; 10, 70, 160, 220, 270, 300, 320] V  VrVec=[10, 20, 40, 50, 70, 80, 100] V  IrVec=[1e-06, 2e-06, 5e-06, 1e-05, 2e-05, 5e-05, .0001] A  Vf=0.6 V  Ron=0.3 Ohm  Goff=1e-8 S  prmExp=ee.enum.diode.expParam.useTwo  I12=[.0137, .545] A  V12=[.6, .7] V  RS=0 Ohm  Tmeas=298.15 K  IS=1e-12 A  ec=1  I1=0.0137 A  V1=0.6 V  N_series=1  N_parallel=1  ZenerEnable=false  Rz=0.3 Ohm  BV=inf V  C_param=ee.enum.diode.capParam.fixed  CJ=0 pF  CJ0=5 pF  Vvec=[.1, 10, 100] V  Cvec=[3.5, 1, .4] pF  VJ=1 V  Mgrad=0.5  FC=0.5  Q_param=ee.enum.diode.recoveryParam.off  iRM=-7.15 A  iF=4 A  didt=-750 A/us  trr_factor=3  trr=115 ns  Qrr=150 nA*s  Vr=-600 V  Ls=150 nH  Erec=0.03 J  TT=50 ns  tau=100 ns  T_param=ee.enum.diode.temperatureParam.off  Tdevice=298.15 K  I1_T2=0.245 A  V1_T2=0.5 V  IS_T2=1.25e-7 A  Tmeas2=125 degC  XTI_param=ee.enum.diode.xtiParam.pn  XTI=3  EG_param=ee.enum.diode.egapParam.material_si  EG=1.11 eV  dBVdT=0 V/K  enable_fault_input=simscape.enum.onoff.off  i_specify=off  i_priority=None  i=0 A  i_nominal_specify=off  i_nominal_value=1  i_nominal_unit=A  v_specify=off  v_priority=None  v=0 V  v_nominal_specify=off  v_nominal_value=1  v_nominal_unit=V  v_capacitor_specify=off  v_capacitor_priority=None  v_capacitor=0 V  v_capacitor_nominal_specify=off  v_capacitor_nominal_value=1  v_capacitor_nominal_unit=V  Qj_specify=off  Qj_priority=High  Qj=0 C  Qj_nominal_specify=off  Qj_nominal_value=1  Qj_nominal_unit=C  i_diode_specify=off  i_diode_priority=None  i_diode=0 A  i_diode_nominal_specify=off  i_diode_nominal_value=1  i_diode_nominal_unit=A  v_diode_specify=off  v_diode_priority=None  v_diode=0 V  v_diode_nominal_specify=off  v_diode_nominal_value=1  v_diode_nominal_unit=V  i_capacitor_specify=off  i_capacitor_priority=None  i_capacitor=0 A  i_capacitor_nominal_specify=off  i_capacitor_nominal_value=1  i_capacitor_nominal_unit=A  power_dissipated_specify=off  power_dissipated_priority=None  power_dissipated=0 W  power_dissipated_nominal_specify=off  power_dissipated_nominal_value=1  power_dissipated_nominal_unit=W  fidelity_level=ee.enum.diode.fidelity.includeChargeDyn  rec_loss_model=ee.enum.diode.reverseRecoveryModel.fixed  ErecVal=0 J  scaleWithIandV=true  ErecMat=zeros(2, 3) J  TjrecVec=[298.15, 398.15] K  IfrecVec=[.1, 1, 10] A  IrecVal=10 A  VrecVal=10 V  tFilter=1 / 1000 / 100 s  thermal_network_parameterization=ee.enum.thermalNetworkTopology.junctionCase  Rth=[0, 10] K/W  Rth_Cauer=[1, 3, 10] K/W  Rth_Foster=[.08, .14, .22, .16] K/W  thermal_mass_parameterization=ee.enum.thermalNetwork.timeconstant  thermal_mass=[0, 1] J/K  thermal_mass_Cauer=[.1, .3, 1] J/K  thermal_mass_Foster=[.001, .005, .05, .5] J/K  thermal_time_constant=[0, 10] s  thermal_time_constant_Cauer=[1, 3, 10] s  thermal_time_constant_Foster=[7e-05, .0007, .01, .08] s  thermal_mass_initial_temperatures=[25, 25] degC  thermal_mass_initial_temperatures_Cauer=[25, 25, 25] degC  junction_thermal_mass=0.01 J/K  Tvec_initial_Foster=[25, 25, 25, 25] degC  no_thermal_network=0  junction_temperature_specify=off  junction_temperature_priority=None  junction_temperature=25 degC  junction_temperature_nominal_specify=off  junction_temperature_nominal_value=1  junction_temperature_nominal_unit=degC
  Electrical Reference : fl_lib/Electrical/Electrical Elements/Electrical Reference
  Mux : Mux  Inputs=12
  PS-Simulink Converter{,1..11} (12 alike) : nesl_utility/PS-Simulink Converter  PhysicalDomain=network_engine_domain  SubClassName=ps_output  LeftPortType=input  RightPortType=output  PseudoPeriodic=off  Frequencies=[]  VectorFormat=inherit  Unit=inherit  AffineConversion=off
  Resistor{,1..11} (12 alike) : fl_lib/Electrical/Electrical Elements/Resistor  R=39 Ohm  i_specify=off  i_priority=None  i=0 A  i_nominal_specify=off  i_nominal_value=1  i_nominal_unit=A  v_specify=off  v_priority=None  v=0 V  v_nominal_specify=off  v_nominal_value=1  v_nominal_unit=V
  Selector : Selector  InputPortWidth=12  IndexOptions=Index vector (dialog)  Indices=1  OutputSizes=1
  Selector1 : Selector  InputPortWidth=12  IndexOptions=Index vector (dialog)  Indices=2  OutputSizes=1
  Selector10 : Selector  InputPortWidth=12  IndexOptions=Index vector (dialog)  Indices=11  OutputSizes=1
  Selector11 : Selector  InputPortWidth=12  IndexOptions=Index vector (dialog)  Indices=12  OutputSizes=1
  Selector2 : Selector  InputPortWidth=12  IndexOptions=Index vector (dialog)  Indices=3  OutputSizes=1
  Selector3 : Selector  InputPortWidth=12  IndexOptions=Index vector (dialog)  Indices=4  OutputSizes=1
  Selector4 : Selector  InputPortWidth=12  IndexOptions=Index vector (dialog)  Indices=5  OutputSizes=1
  Selector5 : Selector  InputPortWidth=12  IndexOptions=Index vector (dialog)  Indices=6  OutputSizes=1
  Selector6 : Selector  InputPortWidth=12  IndexOptions=Index vector (dialog)  Indices=7  OutputSizes=1
  Selector7 : Selector  InputPortWidth=12  IndexOptions=Index vector (dialog)  Indices=8  OutputSizes=1
  Selector8 : Selector  InputPortWidth=12  IndexOptions=Index vector (dialog)  Indices=9  OutputSizes=1
  Selector9 : Selector  InputPortWidth=12  IndexOptions=Index vector (dialog)  Indices=10  OutputSizes=1
  Simulink-PS Converter{,1..11} (12 alike) : nesl_utility/Simulink-PS Converter  PhysicalDomain=network_engine_domain  SubClassName=ps_input  LeftPortType=input  RightPortType=output  PseudoPeriodic=off  Frequencies=[]  NoiseDistribution=none  NoiseParameters=[]  Unit=1  AffineConversion=off  FilteringAndDerivatives=provide  SimscapeFilterOrder=1  InputFilterTimeConstant=0.001  UdotUserProvided=0
  Switch{,1..11} (12 alike) : fl_lib/Electrical/Electrical Elements/Switch  R_closed=0.01 Ohm  G_open=1e-8 1/Ohm  Threshold=0.5  i_specify=off  i_priority=None  i=0 A  i_nominal_specify=off  i_nominal_value=1  i_nominal_unit=A  v_specify=off  v_priority=None  v=0 V  v_nominal_specify=off  v_nominal_value=1  v_nominal_unit=V
  Voltage Sensor{,1..11} (12 alike) : fl_lib/Electrical/Electrical Sensors/Voltage Sensor
  Connection Port : PMIOPort  Side=Right
  Connection Port1 : PMIOPort  Port=2  Side=Right
  Connection Port2 : PMIOPort  Port=3  Side=Right
  Connection Port3 : PMIOPort  Port=4  Side=Right
  Connection Port4 : PMIOPort  Port=5  Side=Right
  Connection Port5 : PMIOPort  Port=6  Side=Right
  Connection Port6 : PMIOPort  Port=7  Side=Right
  Connection Port7 : PMIOPort  Port=8  Side=Right
  Connection Port8 : PMIOPort  Port=9  Side=Right
  Connection Port9 : PMIOPort  Port=10  Side=Right
  Connection Port10 : PMIOPort  Port=11  Side=Right
  Connection Port11 : PMIOPort  Port=12  Side=Right
  Connection Port12 : PMIOPort  Port=13  Side=Right
  Vmod : Outport
  wires:
  PS-Simulink Converter/1 -> Data Type Conversion/1
  PS-Simulink Converter1/1 -> Data Type Conversion1/1
  PS-Simulink Converter2/1 -> Data Type Conversion2/1
  PS-Simulink Converter3/1 -> Data Type Conversion3/1
  PS-Simulink Converter4/1 -> Data Type Conversion4/1
  PS-Simulink Converter5/1 -> Data Type Conversion5/1
  PS-Simulink Converter6/1 -> Data Type Conversion6/1
  PS-Simulink Converter7/1 -> Data Type Conversion7/1
  PS-Simulink Converter8/1 -> Data Type Conversion8/1
  PS-Simulink Converter9/1 -> Data Type Conversion9/1
  PS-Simulink Converter10/1 -> Data Type Conversion10/1
  PS-Simulink Converter11/1 -> Data Type Conversion11/1
  Data Type Conversion/1 -> Mux/1
  Data Type Conversion1/1 -> Mux/2
  Data Type Conversion2/1 -> Mux/3
  Data Type Conversion3/1 -> Mux/4
  Data Type Conversion4/1 -> Mux/5
  Data Type Conversion5/1 -> Mux/6
  Data Type Conversion6/1 -> Mux/7
  Data Type Conversion7/1 -> Mux/8
  Data Type Conversion8/1 -> Mux/9
  Data Type Conversion9/1 -> Mux/10
  Data Type Conversion10/1 -> Mux/11
  Data Type Conversion11/1 -> Mux/12
  Bal_Cmd/1 -> Selector/1, Selector2/1, Selector3/1, Selector4/1, Selector5/1, Selector10/1, Selector11/1, Selector9/1, Selector8/1, Selector7/1, Selector6/1, Selector1/1
  Mux/1 -> Vmod/1
  Selector/1 -> Cast To Double/1
  Cast To Double/1 -> Simulink-PS Converter/1
  Cast To Double1/1 -> Simulink-PS Converter1/1
  Selector1/1 -> Cast To Double1/1
  Selector2/1 -> Cast To Double2/1
  Cast To Double2/1 -> Simulink-PS Converter2/1
  Selector3/1 -> Cast To Double3/1
  Cast To Double3/1 -> Simulink-PS Converter3/1
  Selector4/1 -> Cast To Double4/1
  Cast To Double4/1 -> Simulink-PS Converter4/1
  Selector5/1 -> Cast To Double5/1
  Cast To Double5/1 -> Simulink-PS Converter5/1
  Selector6/1 -> Cast To Double6/1
  Cast To Double6/1 -> Simulink-PS Converter6/1
  Cast To Double7/1 -> Simulink-PS Converter7/1
  Selector7/1 -> Cast To Double7/1
  Selector8/1 -> Cast To Double8/1
  Cast To Double8/1 -> Simulink-PS Converter8/1
  Selector9/1 -> Cast To Double9/1
  Cast To Double9/1 -> Simulink-PS Converter9/1
  Cast To Double10/1 -> Simulink-PS Converter10/1
  Selector10/1 -> Cast To Double10/1
  Cast To Double11/1 -> Simulink-PS Converter11/1
  Selector11/1 -> Cast To Double11/1
  connections:
  Connection Port/RConn1 -- Voltage Sensor/LConn1 -- Resistor/LConn1
  Connection Port1/RConn1 -- Switch/RConn2 -- Resistor1/LConn1 -- Voltage Sensor/RConn2 -- Voltage Sensor1/LConn1
  Connection Port2/RConn1 -- Voltage Sensor1/RConn2 -- Voltage Sensor2/LConn1 -- Resistor2/LConn1 -- Switch1/RConn2
  Connection Port4/RConn1 -- Switch3/RConn2 -- Resistor4/LConn1 -- Voltage Sensor4/LConn1 -- Voltage Sensor3/RConn2
  Connection Port5/RConn1 -- Switch4/RConn2 -- Resistor5/LConn1 -- Voltage Sensor4/RConn2 -- Voltage Sensor5/LConn1
  Voltage Sensor7/LConn1 -- Voltage Sensor6/RConn2 -- Resistor7/LConn1 -- Switch6/RConn2 -- Connection Port7/RConn1
  Voltage Sensor7/RConn2 -- Resistor8/LConn1 -- Switch7/RConn2 -- Connection Port8/RConn1 -- Voltage Sensor8/LConn1
  Connection Port12/RConn1 -- Switch11/RConn2 -- Electrical Reference/LConn1 -- Voltage Sensor11/RConn2
  Voltage Sensor/RConn1 -- PS-Simulink Converter/LConn1
  PS-Simulink Converter1/LConn1 -- Voltage Sensor1/RConn1
  PS-Simulink Converter2/LConn1 -- Voltage Sensor2/RConn1
  Voltage Sensor3/RConn1 -- PS-Simulink Converter3/LConn1
  Voltage Sensor4/RConn1 -- PS-Simulink Converter4/LConn1
  Voltage Sensor5/RConn1 -- PS-Simulink Converter5/LConn1
  PS-Simulink Converter6/LConn1 -- Voltage Sensor6/RConn1
  PS-Simulink Converter7/LConn1 -- Voltage Sensor7/RConn1
  PS-Simulink Converter8/LConn1 -- Voltage Sensor8/RConn1
  PS-Simulink Converter9/LConn1 -- Voltage Sensor9/RConn1
  PS-Simulink Converter10/LConn1 -- Voltage Sensor10/RConn1
  PS-Simulink Converter11/LConn1 -- Voltage Sensor11/RConn1
  Diode/LConn1 -- Resistor/RConn1
  Diode/RConn1 -- Switch/LConn1
  Resistor1/RConn1 -- Diode1/LConn1
  Diode1/RConn1 -- Switch1/LConn1
  Diode2/LConn1 -- Resistor2/RConn1
  Diode2/RConn1 -- Switch2/LConn1
  Voltage Sensor3/LConn1 -- Resistor3/LConn1 -- Switch2/RConn2 -- Connection Port3/RConn1 -- Voltage Sensor2/RConn2
  Resistor3/RConn1 -- Diode3/LConn1
  Diode3/RConn1 -- Switch3/LConn1
  Resistor4/RConn1 -- Diode4/LConn1
  Diode4/RConn1 -- Switch4/LConn1
  Voltage Sensor5/RConn2 -- Resistor6/LConn1 -- Switch5/RConn2 -- Connection Port6/RConn1 -- Voltage Sensor6/LConn1
  Resistor5/RConn1 -- Diode5/LConn1
  Diode5/RConn1 -- Switch5/LConn1
  Resistor6/RConn1 -- Diode6/LConn1
  Switch6/LConn1 -- Diode6/RConn1
  Resistor7/RConn1 -- Diode7/LConn1
  Diode7/RConn1 -- Switch7/LConn1
  Voltage Sensor8/RConn2 -- Resistor9/LConn1 -- Switch8/RConn2 -- Connection Port9/RConn1 -- Voltage Sensor9/LConn1
  Resistor8/RConn1 -- Diode8/LConn1
  Diode8/RConn1 -- Switch8/LConn1
  Voltage Sensor9/RConn2 -- Voltage Sensor10/LConn1 -- Resistor10/LConn1 -- Switch9/RConn2 -- Connection Port10/RConn1
  Resistor9/RConn1 -- Diode9/LConn1
  Diode9/RConn1 -- Switch9/LConn1
  Voltage Sensor10/RConn2 -- Resistor11/LConn1 -- Switch10/RConn2 -- Connection Port11/RConn1 -- Voltage Sensor11/LConn1
  Resistor10/RConn1 -- Diode10/LConn1
  Diode10/RConn1 -- Switch10/LConn1
  Diode11/RConn1 -- Switch11/LConn1
  Diode11/LConn1 -- Resistor11/RConn1
  Simulink-PS Converter/RConn1 -- Switch/RConn1
  Simulink-PS Converter1/RConn1 -- Switch1/RConn1
  Simulink-PS Converter2/RConn1 -- Switch2/RConn1
  Simulink-PS Converter3/RConn1 -- Switch3/RConn1
  Simulink-PS Converter11/RConn1 -- Switch11/RConn1
  Simulink-PS Converter10/RConn1 -- Switch10/RConn1
  Simulink-PS Converter9/RConn1 -- Switch9/RConn1
  Simulink-PS Converter8/RConn1 -- Switch8/RConn1
  Simulink-PS Converter7/RConn1 -- Switch7/RConn1
  Simulink-PS Converter6/RConn1 -- Switch6/RConn1
  Simulink-PS Converter5/RConn1 -- Switch5/RConn1
  Simulink-PS Converter4/RConn1 -- Switch4/RConn1
